simulink model "sldv_property1"  (R2015b)
settings: Solver=FixedStepDiscrete  SolverMode=SingleTasking  StartTime=0.0  StopTime=10.0  RelTol=1e-3
undefined symbols (not defined in the file): sldvsubsys
Description:
  | Model Coverage Test Generation
settings Model: Creator=The MathWorks Inc.  LastModifiedBy=amatsumo
settings DataIOCC: SaveFormat=Array  SignalLoggingSaveFormat=ModelDataLogs  SaveOutput=off  SignalLogging=off  SaveTime=off
settings OptimizationCC: BlockReduction=off  ConditionallyExecuteInputs=off  DefaultParameterBehavior=Inlined  ExpressionDepthLimit=2147483647  InitFltsAndDblsToZero=on  EfficientMapNaN2IntZero=off
settings DebuggingCC: AlgebraicLoopMsg=error  SaveWithParameterizedLinksMsg=none  UnderspecifiedInitializationDetection=Classic  MergeDetectMultiDrivingBlocksExec=none  SignalResolutionControl=TryResolveAllWithWarning  SolverPrmCheckMsg=warning  SingleTaskRateTransMsg=error  FcnCallInpInsideContextMsg=UseLocalSettings  StateNameClashWarn=warning
settings HardwareCC: ProdBitPerPointer=32  ProdLargestAtomicFloat=None  ProdIntDivRoundTo=Undefined  ProdEndianess=Unspecified  ProdWordSize=32  ProdHWDeviceType=ASIC/FPGA->ASIC/FPGA  ProdEqTarget=off
settings SFSimCC: SimParseCustomCode=off
settings GRTTargetCC: TargetFcnLib=ansi_tfl_tmw.mat  GeneratePreprocessorConditionals=Disable all  CombineOutputUpdateFcns=off  GRTInterface=on
settings ConfigComp: RecordCoverage=on  CovModelRefEnable=Off  CovSFcnEnable=off  DVMaxProcessTime=60  DVDisplayUnsatisfiableObjectives=on  DVAutomaticStubbing=off  DVMakeOutputFilesUnique=off  DVParameters=on  DVModelCoverageObjectives=MCDC  DVMaxTestCaseSteps=500  DVTestSuiteOptimization=CombinedObjectives  DVAssertions=EnableAll  DVProofAssumptions=EnableAll  DVDetectActiveLogic=on  DVSaveHarnessModel=on  DVModelReferenceHarness=on  DVSaveReport=on  DVActiveTab=4

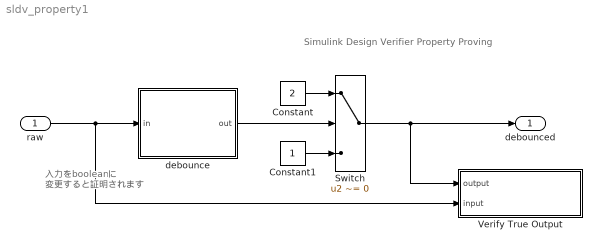
== system sldv_property1 ==
  note: Simulink Design Verifier
      | Property Proving
  note: 入力をbooleanに
      | 変更すると証明されます
  raw : Inport  OutDataTypeStr=uint8  Interpolate=off
  Constant : Constant  Value=2  OutDataTypeStr=uint8
  Constant1 : Constant  OutDataTypeStr=uint8
  Switch : Switch  Criteria=u2 ~= 0
  Verify True Output : Subsystem  Tag=VerificationSubsystem  DisableCoverage=on  LoadFcn=sldvsubsys('check')  TreatAsAtomicUnit=on  SimViewingDevice=on  mask(VerificationSubsystem){}
      mask init:
      | sldvsubsys('maskInit');
      settings: CopyFcn=sldvsubsys('copy');
      settings: PreSaveFcn=|
      | set_param(gcb,'SimViewingDevice','on');
      | sldvsubsys('check');
      mask Display: image(imread('sldvicon_versubsys.png','BackGroundColor',[1 1 1]),'center');
  debounce : Stateflow chart  TreatAsAtomicUnit=on
  debounced : Outport  OutDataTypeStr=uint8
  wires:
  raw/1 -> debounce/1(in), Verify True Output/2(input)
  debounce/1(out) -> Switch/2
  Switch/1 -> debounced/1, Verify True Output/1(output)
  Constant/1 -> Switch/1
  Constant1/1 -> Switch/3

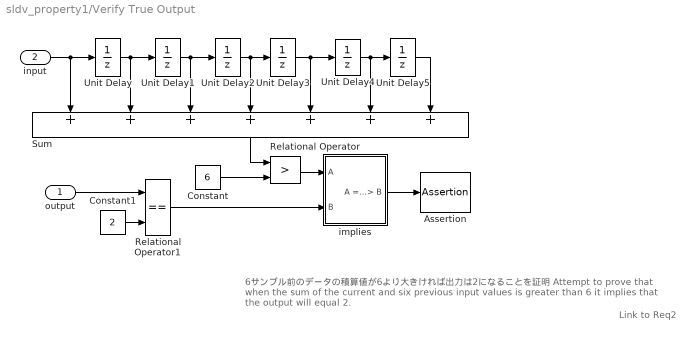
== system sldv_property1/Verify True Output ==
  note: 6サンプル前のデータの積算値が6より大きければ出力は2になることを証明
      | Attempt to prove that when the sum of the current and six previous input
      | values is greater than 6 it implies that the output will equal 2.
  note: Link to Req2
  output : Inport
  input : Inport  Port=2
  Assertion : Assertion
  Constant : Constant  Value=6  OutDataTypeStr=uint8
  Constant1 : Constant  Value=2  OutDataTypeStr=uint8
  Relational Operator : RelationalOperator  Operator=>  OutDataTypeStr=boolean
  Relational Operator1 : RelationalOperator  Operator===  OutDataTypeStr=boolean
  Sum : Sum  Inputs=+++++++
  Unit Delay{,1..5} (6 alike) : UnitDelay  SampleTime=-1
  implies : Subsystem
  wires:
  Unit Delay5/1 -> Sum/7
  implies/1(A ==> B) -> Assertion/1
  Relational Operator1/1 -> implies/2(B)
  Relational Operator/1 -> implies/1(A)
  output/1 -> Relational Operator1/1
  Constant1/1 -> Relational Operator1/2
  Constant/1 -> Relational Operator/2
  Sum/1 -> Relational Operator/1
  Unit Delay4/1 -> Unit Delay5/1, Sum/6
  Unit Delay3/1 -> Sum/5, Unit Delay4/1
  Unit Delay2/1 -> Sum/4, Unit Delay3/1
  Unit Delay1/1 -> Sum/3, Unit Delay2/1
  Unit Delay/1 -> Sum/2, Unit Delay1/1
  input/1 -> Sum/1, Unit Delay/1

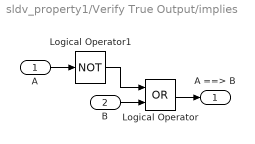
== system sldv_property1/Verify True Output/implies ==
  A : Inport
  B : Inport  Port=2
  Logical Operator : Logic  Operator=OR  AllPortsSameDT=off  OutDataTypeStr=boolean
  Logical Operator1 : Logic  Operator=NOT  AllPortsSameDT=off  OutDataTypeStr=boolean
  A ==> B : Outport
  wires:
  B/1 -> Logical Operator/2
  Logical Operator/1 -> A ==> B/1
  A/1 -> Logical Operator1/1
  Logical Operator1/1 -> Logical Operator/1

== stateflow chart sldv_property1/debounce ==
  settings: updateMethod=DISCRETE  sampleTime=0.01  stateMachineType=MOORE_MACHINE  executeAtInitialization=1  initializeOutput=1
  state Off
    out = 0;
  state On
    out = 1;
  (default) -> Off
  Off -> On : [in==1]
  On -> Off : [in==0]
  data: in input; out output boolean
